simulink model "SEDC_Motor_Model"  (R2023b)
settings: Solver=VariableStepAuto  StartTime=0.0  StopTime=.02  MaxStep=1e-6
values from neighbouring files (symbols this model uses):
  B = 0.01    [SEDC_Model_Init.m]
  J = 5    [SEDC_Model_Init.m]
  Kphi = 1.6    [SEDC_Model_Init.m]
  La = 0.1    [SEDC_Model_Init.m]
  Ra = 0.5    [SEDC_Model_Init.m]
  TL = 20    [SEDC_Model_Init.m]
libraries: spsThyristorLib x4, spsVoltageMeasurementLib x3, spsSeriesRLCBranchLib x2, simulink x2, spsACVoltageSourceLib x1, dspswit3 x1, spsUniversalBridgeLib x1, sps_lib x1
settings Model: Creator=Abdelrhman Shaban  LastModifiedBy=ascom
settings OptimizationCC: ReuseModelBlockBuffer=off

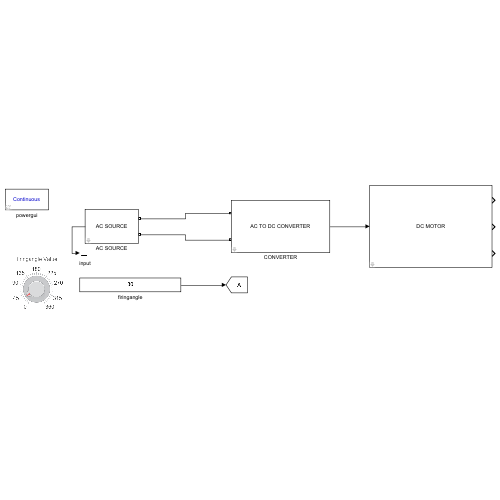
[thumbnail: Simulink's stored preview of the top-level diagram]
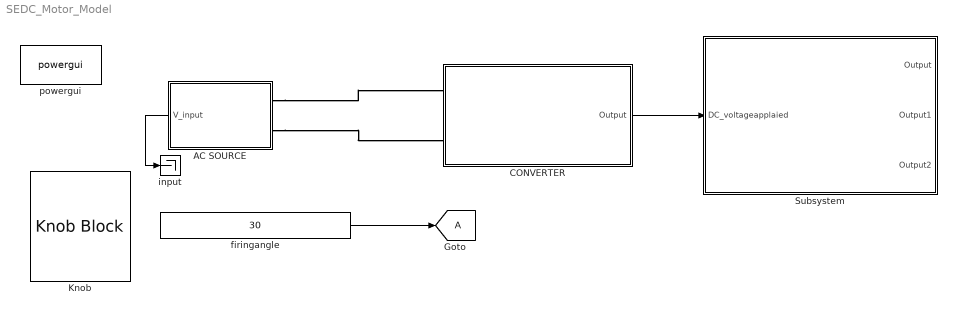
== system SEDC_Motor_Model ==
  AC SOURCE : Subsystem
      mask DialogControl ACsource Prompt: source
      mask DialogControl Container3 Prompt: voltage
      mask DialogControl Container4 Prompt: frequancy
      mask Display: disp('AC SOURCE');
  CONVERTER : Subsystem
      mask DialogControl DescTextVar Prompt: CONVERTER
      mask DialogControl firingangle Prompt: FIRINGANGLE
      mask DialogControl zcangle Prompt: ZEROCROSSANGLE
      mask Display: disp('AC TO DC CONVERTER');
  Goto : Goto  TagVisibility=global
  Knob : KnobBlock  ScaleMax=360
  Subsystem : Subsystem
      mask Display: disp('DC MOTOR');
  firingangle : Constant  Value=30
  input : Terminator
  powergui : sps_lib/powergui  Priority=1  SimulationMode=Continuous  SampleTime=50e-6  frequency=60  Iterations=50  frequencyindice=50  Pbase=100e6  ErrMax=1e-4  UnitsV=kV  UnitsW=MW  buscounter=0  FunctionMessages=off  echomessages=off  EnableUseOfTLC=off  CurrentSourceSwitches=off  DisableSnubberDevices=off  DisableRonSwitches=off  DisableVfSwitches=off  DisplayEquations=off  AutomaticDiscreteSolvers=off  SolverType=Tustin/Backward Euler (TBE)  Interpol=off  ExternalGateDelay=off  methode=off  Ts=100  x0status=blocks  SPID=on  SwTol=0  HookPort=off  NonlinearTolerance=1e-4  nMaxIteration=100  ContinueOnMaxIteration=off  RestoreLinks=warning  ResistiveCurrentMeasurement=off  Frange=[0:2:500]  Ylog=off  Xlog=on  ShowGrid=off  save=off  variable=ZData  structure=0  ZoomFFT=off  StartTime=0.0  cycles=1  DisplayStyle=1  fundamental=60  FreqAxis=off  MaxFrequency=1000  frequencyindicesteady=1  RmsSteady=1  display=off
  wires:
  AC SOURCE/1(V_input) -> input/1
  firingangle/1 -> Goto/1
  CONVERTER/1(Output) -> Subsystem/1(DC_voltageapplaied)
  connections:
  AC SOURCE/LConn1 -- CONVERTER/LConn1
  AC SOURCE/LConn2 -- CONVERTER/LConn2

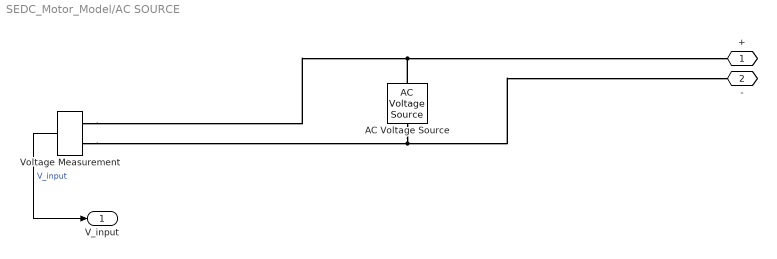
== system SEDC_Motor_Model/AC SOURCE ==
  AC Voltage Source : spsACVoltageSourceLib/AC Voltage Source  Amplitude=220  Phase=0  Frequency=50  SampleTime=0  Measurements=None  BusType=swing  Pref=10e3  Qref=0  Qmin=-inf  Qmax=+inf
  Voltage Measurement : spsVoltageMeasurementLib/Voltage Measurement  PhasorSimulation=off  OutputType=Complex  PSBequivalent=0
  + : PMIOPort  Side=Left
  - : PMIOPort  Port=2  Side=Left
  V_input : Outport
  wires:
  Voltage Measurement/1 -> V_input/1  "V_input"
  connections:
  Voltage Measurement/LConn1 -- AC Voltage Source/RConn1 -- +/RConn1
  Voltage Measurement/LConn2 -- AC Voltage Source/LConn1 -- -/RConn1

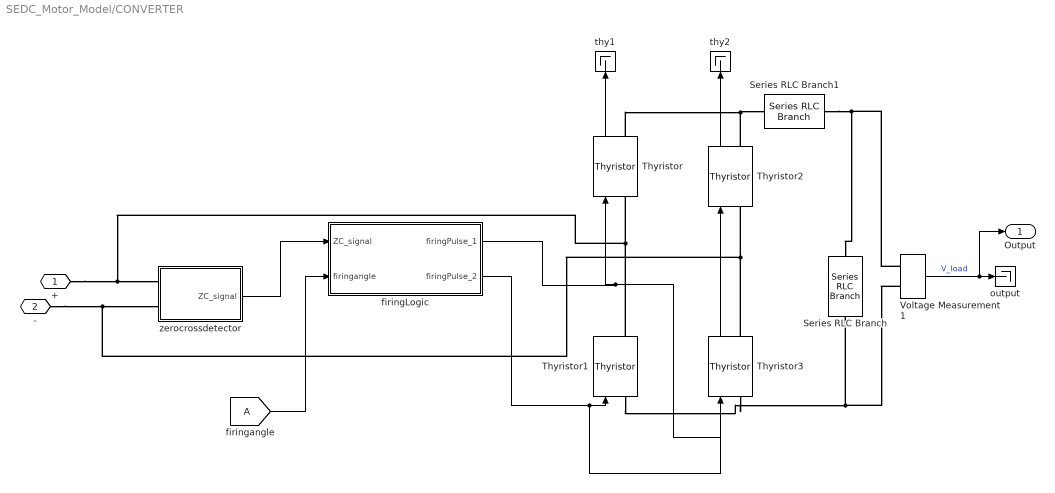
== system SEDC_Motor_Model/CONVERTER ==
  Series RLC Branch : spsSeriesRLCBranchLib/Series RLC Branch  LConnTagsString=__new0  RConnTagsString=__new0  BranchType=C  Resistance=50  Inductance=1e-3  SetiL0=off  InitialCurrent=0  Capacitance=1e-6  Setx0=off  InitialVoltage=0  Measurements=None
  Series RLC Branch1 : spsSeriesRLCBranchLib/Series RLC Branch  LConnTagsString=__new0  RConnTagsString=__new0  BranchType=R  Resistance=40  Inductance=1e-3  SetiL0=off  InitialCurrent=0  Capacitance=1e-6  Setx0=off  InitialVoltage=0  Measurements=None
  Thyristor{,1..3} (4 alike) : spsThyristorLib/Thyristor  Ron=0.001  Lon=0  Vf=0.8  IC=0  Rs=500  Cs=250e-9  Measurements=on
  Voltage Measurement1 : spsVoltageMeasurementLib/Voltage Measurement  PhasorSimulation=off  OutputType=Complex  PSBequivalent=0
  firingLogic : Subsystem
  firingangle : From  TagVisibility=global
  output : Terminator
  thy1 : Terminator
  thy2 : Terminator
  zerocrossdetector : Subsystem
  + : PMIOPort  Side=Left
  - : PMIOPort  Port=2  Side=Left
  Output : Outport
  wires:
  zerocrossdetector/1(ZC_signal) -> firingLogic/1(ZC_signal)
  Voltage Measurement1/1 -> Output/1, output/1  "V_load"
  firingLogic/1(firingPulse_1) -> Thyristor3/1, Thyristor/1
  firingLogic/2(firingPulse_2) -> Thyristor1/1, Thyristor2/1
  Thyristor/1 -> thy1/1
  Thyristor2/1 -> thy2/1
  firingangle/1 -> firingLogic/2(firingangle)
  connections:
  Voltage Measurement1/LConn1 -- Series RLC Branch/LConn1 -- Series RLC Branch1/LConn1
  Voltage Measurement1/LConn2 -- Series RLC Branch/RConn1 -- Thyristor1/LConn1 -- Thyristor3/LConn1
  Thyristor/RConn1 -- Series RLC Branch1/RConn1 -- Thyristor2/RConn1
  Thyristor1/RConn1 -- zerocrossdetector/LConn1 -- +/RConn1 -- Thyristor/LConn1
  Thyristor3/RConn1 -- zerocrossdetector/LConn2 -- -/RConn1 -- Thyristor2/LConn1

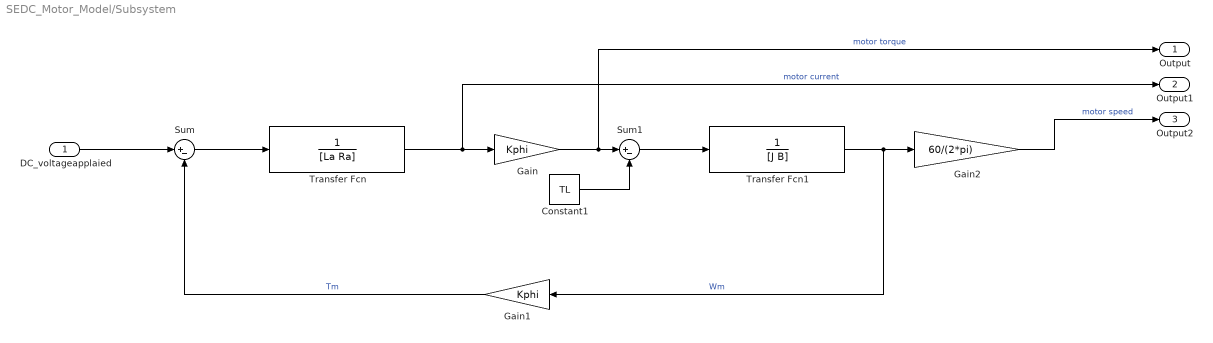
== system SEDC_Motor_Model/Subsystem ==
  DC_voltageapplaied : Inport
  Constant1 : Constant  Value=TL
  Gain : Gain  Gain=Kphi
  Gain1 : Gain  Gain=Kphi
  Gain2 : Gain  Gain=60/(2*pi)
  Sum : Sum  Inputs=|+-
  Sum1 : Sum  Inputs=|+-
  Transfer Fcn : TransferFcn  Denominator=[La Ra]
  Transfer Fcn1 : TransferFcn  Denominator=[J B]
  Output : Outport
  Output1 : Outport  Port=2
  Output2 : Outport  Port=3
  wires:
  Sum1/1 -> Transfer Fcn1/1
  Gain/1 -> Output/1, Sum1/1  "motor torque"
  Transfer Fcn1/1 -> Gain1/1, Gain2/1  "Wm"
  Constant1/1 -> Sum1/2
  Transfer Fcn/1 -> Output1/1, Gain/1  "motor current"
  Gain1/1 -> Sum/2  "Tm"
  Gain2/1 -> Output2/1  "motor speed"
  Sum/1 -> Transfer Fcn/1
  DC_voltageapplaied/1 -> Sum/1

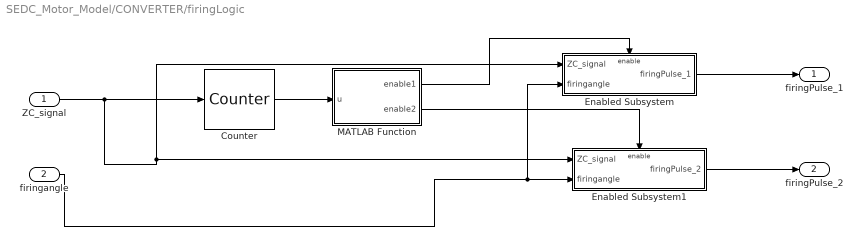
== system SEDC_Motor_Model/CONVERTER/firingLogic ==
  ZC_signal : Inport
  firingangle : Inport  Port=2
  Counter : dspswit3/Counter  Direction=Up  CountEvent=Rising edge  CounterSize=User defined  MaxCount=255  InitialCount=0  Output=Count  HitValue=32  ResetInput=off  SamplesPerFrame=1  Ts=1  CntDtype=double  HitDtype=Logical
  Enabled Subsystem : Subsystem  TreatAsAtomicUnit=on
  Enabled Subsystem1 : Subsystem  TreatAsAtomicUnit=on
  MATLAB Function : MATLAB Function  TreatAsAtomicUnit=on
  firingPulse_1 : Outport
  firingPulse_2 : Outport  Port=2
  wires:
  ZC_signal/1 -> Enabled Subsystem/1(ZC_signal), Enabled Subsystem1/1(ZC_signal), Counter/1
  Counter/1 -> MATLAB Function/1(u)
  MATLAB Function/1(enable1) -> Enabled Subsystem/Enable
  MATLAB Function/2(enable2) -> Enabled Subsystem1/Enable
  firingangle/1 -> Enabled Subsystem/2(firingangle), Enabled Subsystem1/2(firingangle)
  Enabled Subsystem/1(firingPulse_1) -> firingPulse_1/1
  Enabled Subsystem1/1(firingPulse_2) -> firingPulse_2/1

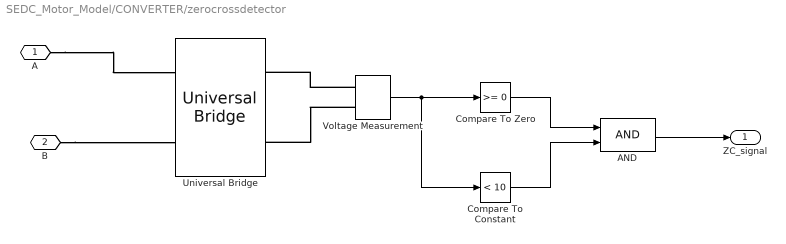
== system SEDC_Motor_Model/CONVERTER/zerocrossdetector ==
  AND : Logic  AllPortsSameDT=off  OutDataTypeStr=boolean
  Compare To Constant : simulink/Logic and Bit Operations/Compare To Constant  relop=<  const=10  OutDataTypeStr=boolean
  Compare To Zero : simulink/Logic and Bit Operations/Compare To Zero  relop=>=  OutDataTypeStr=boolean
  Universal Bridge : spsUniversalBridgeLib/Universal Bridge  Arms=2  SnubberResistance=1e5  SnubberCapacitance=inf  Device=Diodes  Ron=1e-3  Lon=0  ForwardVoltages="[  0  0  ]"  ForwardVoltage=0  GTOparameters=[ 10e-6 , 20e-6 ]  IGBTparameters=[ 1e-6 , 2e-6 ]  Measurements=None  Measurements_2=None  converterType=Rectifier
  Voltage Measurement : spsVoltageMeasurementLib/Voltage Measurement  PhasorSimulation=off  OutputType=Complex  PSBequivalent=0
  A : PMIOPort  Side=Left
  B : PMIOPort  Port=2  Side=Left
  ZC_signal : Outport
  wires:
  Voltage Measurement/1 -> Compare To Constant/1, Compare To Zero/1
  Compare To Constant/1 -> AND/2
  Compare To Zero/1 -> AND/1
  AND/1 -> ZC_signal/1
  connections:
  A/RConn1 -- Universal Bridge/LConn1
  B/RConn1 -- Universal Bridge/LConn2
  Voltage Measurement/LConn1 -- Universal Bridge/RConn1
  Voltage Measurement/LConn2 -- Universal Bridge/RConn2

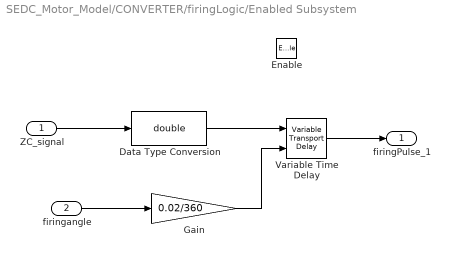
== system SEDC_Motor_Model/CONVERTER/firingLogic/Enabled Subsystem ==
  ZC_signal : Inport
  firingangle : Inport  Port=2
  Enable : EnablePort
  Data Type Conversion : DataTypeConversion  OutDataTypeStr=double  SaturateOnIntegerOverflow=off  RndMeth=Floor
  Gain : Gain  Gain=0.02/360
  Variable Time Delay : VariableTransportDelay  MaximumDelay=10
  firingPulse_1 : Outport
  wires:
  firingangle/1 -> Gain/1
  Gain/1 -> Variable Time Delay/2
  Variable Time Delay/1 -> firingPulse_1/1
  Data Type Conversion/1 -> Variable Time Delay/1
  ZC_signal/1 -> Data Type Conversion/1

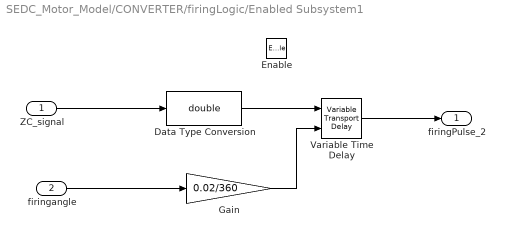
== system SEDC_Motor_Model/CONVERTER/firingLogic/Enabled Subsystem1 ==
  ZC_signal : Inport
  firingangle : Inport  Port=2
  Enable : EnablePort
  Data Type Conversion : DataTypeConversion  OutDataTypeStr=double  SaturateOnIntegerOverflow=off  RndMeth=Floor
  Gain : Gain  Gain=0.02/360
  Variable Time Delay : VariableTransportDelay  MaximumDelay=10
  firingPulse_2 : Outport
  wires:
  Data Type Conversion/1 -> Variable Time Delay/1
  Gain/1 -> Variable Time Delay/2
  ZC_signal/1 -> Data Type Conversion/1
  firingangle/1 -> Gain/1
  Variable Time Delay/1 -> firingPulse_2/1

== matlab function SEDC_Motor_Model/CONVERTER/firingLogic/MATLAB Function ==
  data: u input; enable1 output; enable2 output
function [enable1,enable2] = fcn(u)
enable1=0;
enable2=0;
if mod(u,2)==0
enable1=1;
enable2=0;
end 
if mod(u,2)==1
enable1=0;
enable2=1;
end
